simulink model "Project"  (R2018a)
settings: Solver=VariableStepAuto  StartTime=0.0  StopTime=0.3  FixedStep=0.02  RelTol=1e-3
libraries: powerlib x10, re_lib x1, powerlib_meascontrol x1
settings Model: Creator=ACER  LastModifiedBy=ACER

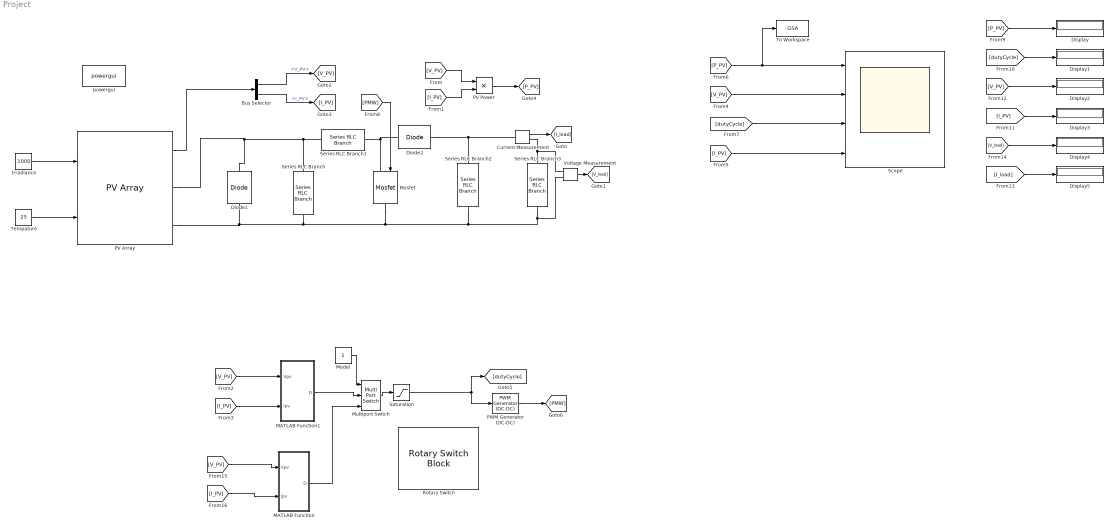
== system Project ==
  Bus Selector : BusSelector  OutputSignals=V_PV,I_PV
  Current Measurement : powerlib/Measurements/Current Measurement  PhasorSimulation=off  OutputType=Complex  PSBequivalent=0
  Diode1 : powerlib/Power Electronics/Diode  Ron=0.001  Lon=0  Vf=0.8  IC=0  UseSnubber=0  Rs=500  Cs=250e-9  Measurements=off
  Diode2 : powerlib/Power Electronics/Diode  Ron=0.001  Lon=0  Vf=0.8  IC=0  UseSnubber=0  Rs=500  Cs=250e-9  Measurements=off
  Display{,1..5} (6 alike) : Display
  Irradiance : Constant  Value=1000
  MATLAB Function : MATLAB Function  TreatAsAtomicUnit=on
  MATLAB Function1 : MATLAB Function  TreatAsAtomicUnit=on
  "Model " : Constant
  Mosfet : powerlib/Power Electronics/Mosfet  Ron=1e-3  Lon=0  Rd=1e-3  Vfd=0  IC=0  Rs=inf  Cs=inf  Measurements=off
  Multiport Switch : MultiPortSwitch  Inputs=2
  PV Array : re_lib/Solar/PV Array  Npar=1  Nser=1  PlotType=array @ 25 deg.C & specified irradiances  S_vec="[ 1000  700  400 ]"  Temp_C_vec="[ 45 25  ]"  ModuleName=User-defined  PlotWhenSelected=off  Pm=55.5  Ncell=20  Voc=21.7  Isc=4.8  Vm=15  Im=3.7  beta_Voc_pc=-0.33641  alpha_Isc_pc=0.102  beta_Voc=-0.073001  alpha_Isc=0.004896  IL=5.1788  I0=4.9208e-11  nI=1.6839  Rsh=15.6707  Rs=1.167  BAL=off  Tc=1e-6  Tfilter=5e-5
  PV Power : Product
  PWM Generator (DC-DC) : powerlib_meascontrol/Pulse & Signal Generators/PWM Generator (DC-DC)  Fsw=10000  Ts=0
  Rotary Switch : RotarySwitchBlock  WebBlockId=82
      settings: Values={{'GSA', 'PSO'}, [1 2]}
  Saturation : Saturate  UpperLimit=1  LowerLimit=0
  Scope : Scope  NumInputPorts=4
  Series RLC Branch : powerlib/Elements/Series RLC Branch  LConnTagsString=__new0  RConnTagsString=__new0  BranchType=C  Resistance=1  Inductance=1e-3  SetiL0=off  InitialCurrent=0  Capacitance=470e-6  Setx0=off  InitialVoltage=0  Measurements=None
  Series RLC Branch1 : powerlib/Elements/Series RLC Branch  LConnTagsString=__new0  RConnTagsString=__new0  BranchType=L  Resistance=1  Inductance=1.2e-3  SetiL0=off  InitialCurrent=0  Capacitance=1e-3  Setx0=off  InitialVoltage=0  Measurements=None
  Series RLC Branch2 : powerlib/Elements/Series RLC Branch  LConnTagsString=__new0  RConnTagsString=__new0  BranchType=C  Resistance=1  Inductance=1e-3  SetiL0=off  InitialCurrent=0  Capacitance=47e-6  Setx0=off  InitialVoltage=0  Measurements=None
  Series RLC Branch3 : powerlib/Elements/Series RLC Branch  LConnTagsString=__new0  RConnTagsString=__new0  BranchType=R  Resistance=58  Inductance=1e-3  SetiL0=off  InitialCurrent=0  Capacitance=1e-3  Setx0=off  InitialVoltage=0  Measurements=None
  Tempature : Constant  Value=25
  To Workspace : ToWorkspace  VariableName=GSA  SaveFormat=Timeseries  SampleTime=-1
  Voltage Measurement : powerlib/Measurements/Voltage Measurement  PhasorSimulation=off  OutputType=Complex  PSBequivalent=0
  powergui : powerlib/powergui  Priority=1  SimulationMode=Discrete  SampleTime=1e-6  frequency=60  Iterations=50  frequencyindice=0  Pbase=100e6  ErrMax=1e-4  UnitsV=kV  UnitsW=MW  buscounter=0  FunctionMessages=off  echomessages=off  EnableUseOfTLC=off  CurrentSourceSwitches=off  DisableSnubberDevices=off  DisableRonSwitches=off  DisableVfSwitches=off  DisplayEquations=off  SolverType=Tustin/Backward Euler (TBE)  Interpol=off  ExternalGateDelay=off  methode=off  Ts=100  x0status=blocks  SPID=off  SwTol=0  HookPort=off  RestoreLinks=warning  ResistiveCurrentMeasurement=off  Frange=[0:2:500]  Ylog=off  Xlog=on  ShowGrid=off  save=off  variable=ZData  structure=0  ZoomFFT=off  StartTime=0.0  cycles=1  DisplayStyle=1  fundamental=60  FreqAxis=off  MaxFrequency=1000  frequencyindicesteady=1  RmsSteady=1  display=off
  wires:
  Irradiance/1 -> PV Array/1
  Tempature/1 -> PV Array/2
  Current Measurement/1 -> [I_load]
  Voltage Measurement/1 -> [V_load]
  PV Array/1 -> Bus Selector/1
  Bus Selector/1 -> [V_PV]  "<V_PV>"
  Bus Selector/2 -> [I_PV]  "<I_PV>"
  [I_PV] -> PV Power/2
  [V_PV] -> PV Power/1
  PV Power/1 -> [P_PV]
  Saturation/1 -> PWM Generator (DC-DC)/1, [dutyCycle]
  PWM Generator (DC-DC)/1 -> [PMW]
  [V_PV] -> Scope/2
  [P_PV] -> To Workspace/1, Scope/1
  [dutyCycle] -> Scope/3
  [I_PV] -> Scope/4
  [PMW] -> Mosfet/1
  [P_PV] -> Display/1
  [dutyCycle] -> Display1/1
  [I_PV] -> Display3/1
  [V_PV] -> Display2/1
  [I_load] -> Display5/1
  [V_load] -> Display4/1
  MATLAB Function1/1(D) -> Multiport Switch/2
  [V_PV] -> MATLAB Function1/1(Vpv)
  [I_PV] -> MATLAB Function1/2(Ipv)
  Multiport Switch/1 -> Saturation/1
  "Model "/1 -> Multiport Switch/1
  [V_PV] -> MATLAB Function/1(Vpv)
  [I_PV] -> MATLAB Function/2(Ipv)
  MATLAB Function/1(D) -> Multiport Switch/3
  connections:
  PV Array/RConn1 -- Series RLC Branch/LConn1 -- Series RLC Branch1/LConn1 -- Diode1/RConn1
  PV Array/RConn2 -- Voltage Measurement/LConn2 -- Series RLC Branch3/RConn1 -- Series RLC Branch2/RConn1 -- Mosfet/RConn1 -- Series RLC Branch/RConn1 -- Diode1/LConn1
  Diode2/LConn1 -- Series RLC Branch1/RConn1 -- Mosfet/LConn1
  Diode2/RConn1 -- Current Measurement/LConn1 -- Series RLC Branch2/LConn1
  Current Measurement/RConn1 -- Voltage Measurement/LConn1 -- Series RLC Branch3/LConn1

== matlab function Project/MATLAB Function1 ==
  settings: updateMethod=DISCRETE
  data: Vpv input; D output; Ipv input
function D = GSA(Vpv,Ipv)
coder.extrinsic('randi')
persistent u;
persistent dcurrent;%store current duty cycle
persistent pbest;%store local best dc for power
persistent force; %store force
persistent acceleration; %store acceleration
persistent mass; % mass
persistent q; %  strength of mass
persistent p; %  power for each particle
persistent p_current; %  power current for each particle
persistent p_min; %  power min for each particle
persistent worse;   %store best worse of each particle 
persistent dc; %store duty cycle ~ position 
persistent v;  %velocity
persistent counter; %delay iteration
persistent iteration;
persistent gbest;%store global best dc for power
%initialization

max_iter = 3000;
if(isempty(counter))
    counter = 0;
    dcurrent = 0.5; 
    gbest = 0.5;
    pbest = zeros(3,1);
    worse = zeros(3,1);
    v = zeros (3,1);
    force = zeros(3,1);
    mass = zeros(3,1);
    q = zeros(3,1);
    p = zeros(3,1);
    p_current = zeros(3,1);
    p_min=zeros(3,1);
   
    acceleration=zeros(3,1);
    u = 0;
    dc = zeros (3,1); 
    iteration = 1;
    
    %initialize position for each particle
        dc(1)=0.69;
        dc(2)= 0.7;
        dc(3)=0.8;
        
end

if(counter >=1 && counter < 3000)
    D=dcurrent;
    counter= counter+1;
    return;
end

if(u>=1 && u<=3)
    p_current(u) = Vpv*Ipv;
    if((Vpv*Ipv)>=p(u))
        p(u) = Vpv*Ipv;
        pbest(u)=dcurrent;
    end
    if(Vpv*Ipv < p_min(u))
        p_min(u) = Vpv*Ipv;
        worse(u) = dcurrent;
    end
end
u=u+1;
if(u==5)
    u=1;
end
if(u >= 1 && u <= 3)
    %Avoid over shooting
    if(iteration < max_iter)
        D=dc(u);
        dcurrent=D;
        counter=1;
    return;
    else
        D = dcurrent;
        return
    end
elseif(u==4)
    iteration = iteration +1;
    [~,i]=max(p);
    gbest=pbest(i);
    D=gbest;
    dcurrent=D;
    counter=1;
     %Calculate strength of mass
    for i = 1:3
     q(i) = (p_current(i) - worse(i))/(pbest(i)-worse(i));
    end
     %Calculate sum of strength of mass

     sum_strength_of_mass = q(1) + q(2) + q(3);
    
    %Calculate mass   
    for i = 1:3
     mass(i) = q(i)/sum_strength_of_mass;
    
    end
    %Calculate force
    alpha = 200;
    G0 = 1;
    G = G0 * exp(-alpha*iteration/max_iter);
    %G = 6.67430 * 10^-13; %gravitational constant
    e = 2.2204*10^-16;
    force(1) = rand()*G*(mass(3)*mass(1)*(dc(3)-dc(1))/(Euclidian_distance(dc(3),dc(1))+e) + mass(2)*mass(1)*(dc(3)-dc(1))/(Euclidian_distance(dc(3),dc(1))+e));
    force(2) = rand()*G*(mass(3)*mass(2)*(dc(3)-dc(2))/(Euclidian_distance(dc(3),dc(2))+e) + mass(1)*mass(2)*(dc(1)-dc(2))/(Euclidian_distance(dc(1),dc(2))+e));
    force(3) = rand()*G*(mass(2)*mass(3)*(dc(2)-dc(3))/(Euclidian_distance(dc(2),dc(3))+e) + mass(1)*mass(3)*(dc(1)-dc(3))/(Euclidian_distance(dc(1),dc(3))+e));
    %Avoid over shooting
    if(iteration == max_iter)
        
        D=dcurrent;
        return;
    end
    %Calculate acceleration 
    for i = 1:3
        acceleration(i) = force(i)/mass(i);
        
    end
    
    for i=1:3
        
     v(i)=updatevelocity(v(i),acceleration(i));
     
     dc(i)=updateduty(dc(i),v(i));
     
    end  
    return;
    
else
    D=0.5;
end
end


function d = Euclidian_distance(d1,d2)
    d = sqrt(d1^2+d2^2);
end


function vfinal=updatevelocity(velocity,acceleration)
    vfinal = rand()*velocity + acceleration;
end

function dfinal=updateduty(d,velocity)
dup=d+velocity;
if(dup>1)
    dfinal=1;
elseif(dup<0.1)
    dfinal=0.1;
else
    dfinal=dup;
end
end

== matlab function Project/MATLAB Function ==
  settings: updateMethod=DISCRETE
  data: Vpv input; D output; Ipv input
function D = PSO(Vpv, Ipv)
    coder.extrinsic('randi')
    persistent localbest globalbest k p dc Pbest Pprev dcurrent u v temp;
    c1 = 1;
    c2 = 2;
    P = Ipv * Vpv;
    if isempty(globalbest)
        k = 0;
        dc = zeros(3,1);
        dc(1)=randi( [5 330])/1000;
        dc(2)=randi( [330 660])/1000;
        dc(3)=randi( [660 995])/1000;
        p = zeros(3,1);
        localbest = zeros(3,1);
        v = zeros(3,1);
        Pbest = Ipv * Vpv;
        Pprev = 0;
        dcurrent = 0.5;
        globalbest = dcurrent;
        u=0;
        temp = 0;
    end
    D=dcurrent;
 
    if (temp < 0)
        temp = temp + 1;
        return;
    end
    if (P > Pbest)
        Pbest = P;        
    end
    if (k < 3000)
        k=k+1;
        return;
    else
        k=0;
    end
    if abs(P - Pprev) < 1
       if abs(P - Pbest) > 15
          dc(1)=randi( [5 330])/1000;
          dc(2)=randi( [330 660])/1000;
          dc(3)=randi( [660 995])/1000;
          v = zeros(3,1);
          localbest = zeros(3,1);
          p = zeros(3,1);
          u= 0;
       end
    end
    
    if(u>=1 && u<=3)
        if(P>p(u))
            p(u)=P;
            localbest(u)=dcurrent;
        end
    end
    
    u=u+1;
    
    if (u > 4)
        u=1;
    end
    if (u == 4)
        [~,idx]=max(p);
        globalbest=localbest(idx);
        D = globalbest;
        dcurrent=D;
        for j=1:3
                v(j)=updatevelocity(c1,c2,v(j),localbest(j),dc(j),globalbest);
                dc(j)=updateduty(dc(j),v(j));
        end
    else
        D=dc(u);
        dcurrent=dc(u);
        Pprev = P;
    end
    
  
end

function vfinal=updatevelocity(c1,c2,velocity,pobest,d,gwbest)
    % PSO Parameters
    vfinal = (0.1*velocity)+(c1*rand(1)*(pobest-d))+(c2*rand(1)*(gwbest-d));
end

function dfinal=updateduty(d,velocity)
    dup=d+velocity;
    if(dup>1)
        dfinal=1;
    elseif(dup<0)
        dfinal=abs(dup);
    else
        dfinal=dup;
    end
end
